simulink model "New_Dstatcom_model"  (R2023a)
settings: Solver=VariableStepAuto  StartTime=0.0  StopTime=0.5  RelTol=1e-3
libraries: spsSeriesRLCBranchLib x10, spsThreePhaseBreakerLib x9, spsThreePhaseSeriesRLCLoadLib x9, spsIGBTDiodeLib x6, spsPower3phInstantaneousLib x3, fuzblock x3, spsThreePhaseVIMeasurementLib x3, spsAlphaBetaZerotodq0Lib x2, spsabctodq0Lib x2, slpidlib x1, simulink x1, spsdq0toabcLib x1
settings Model: Creator=Lenovo  LastModifiedBy=Deepak

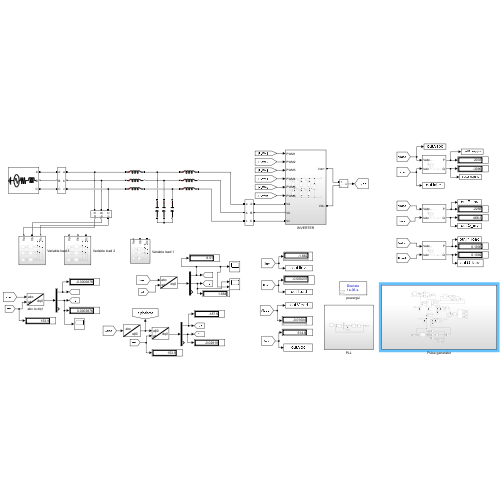
[thumbnail: Simulink's stored preview of the top-level diagram]
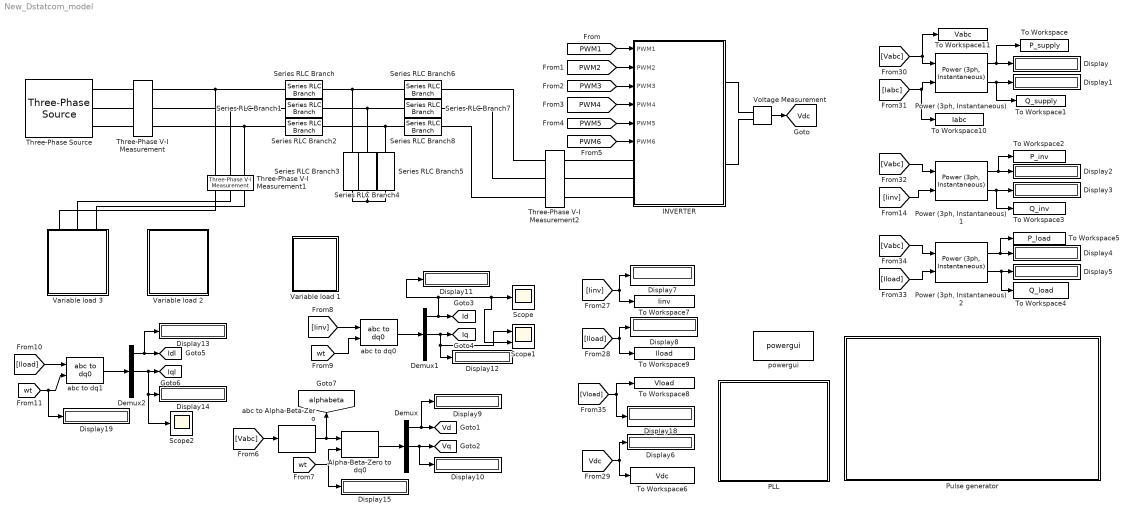
== system New_Dstatcom_model ==
  Alpha-Beta-Zero to dq0 : spsAlphaBetaZerotodq0Lib/Alpha-Beta-Zero to dq0  Alignment=90 degrees behind phase A axis
  Demux : Demux  Outputs=3
  Demux1 : Demux  Outputs=3
  Demux2 : Demux  Outputs=3
  Display{,1..15,18..19} (18 alike) : Display
  INVERTER : Subsystem
  PLL : Subsystem
  "Power (3ph, Instantaneous)" : spsPower3phInstantaneousLib/Power (3ph, Instantaneous)
  "Power (3ph, Instantaneous)1" : spsPower3phInstantaneousLib/Power (3ph, Instantaneous)
  "Power (3ph, Instantaneous)2" : spsPower3phInstantaneousLib/Power (3ph, Instantaneous)
  Pulse generator : Subsystem
  Scope : Scope
  Scope1 : Scope  NumInputPorts=2
  Scope2 : Scope
  Series RLC Branch{,1..2,6..8} (6 alike) : spsSeriesRLCBranchLib/Series RLC Branch  LConnTagsString=__new0  RConnTagsString=__new0  BranchType=L  Resistance=1  Inductance=500e-6  SetiL0=off  InitialCurrent=0  Capacitance=1e-6  Setx0=off  InitialVoltage=0  Measurements=None
  Series RLC Branch3 : spsSeriesRLCBranchLib/Series RLC Branch  LConnTagsString=__new0  RConnTagsString=__new0  BranchType=C  Resistance=1  Inductance=500e-6  SetiL0=off  InitialCurrent=0  Capacitance=100e-6  Setx0=off  InitialVoltage=0  Measurements=None
  Series RLC Branch4 : spsSeriesRLCBranchLib/Series RLC Branch  LConnTagsString=__new0  RConnTagsString=__new0  BranchType=C  Resistance=1  Inductance=500e-6  SetiL0=off  InitialCurrent=0  Capacitance=100e-6  Setx0=off  InitialVoltage=0  Measurements=None
  Series RLC Branch5 : spsSeriesRLCBranchLib/Series RLC Branch  LConnTagsString=__new0  RConnTagsString=__new0  BranchType=C  Resistance=1  Inductance=500e-6  SetiL0=off  InitialCurrent=0  Capacitance=100e-6  Setx0=off  InitialVoltage=0  Measurements=None
  Three-Phase V-I Measurement : spsThreePhaseVIMeasurementLib/Three-Phase V-I Measurement  VoltageMeasurement=phase-to-ground  SetLabelV=on  LabelV=Vabc  Vpu=off  VpuLL=off  CurrentMeasurement=yes  SetLabelI=on  LabelI=Iabc  Ipu=off  Pbase=100e6  Vbase=500e3  OutputType=Complex  PhasorSimulation=off  PSBequivalent=0
  Three-Phase V-I Measurement1 : spsThreePhaseVIMeasurementLib/Three-Phase V-I Measurement  VoltageMeasurement=phase-to-ground  SetLabelV=on  LabelV=Vload  Vpu=off  VpuLL=off  CurrentMeasurement=yes  SetLabelI=on  LabelI=Iload  Ipu=off  Pbase=100e6  Vbase=500e3  OutputType=Complex  PhasorSimulation=off  PSBequivalent=0
  Three-Phase V-I Measurement2 : spsThreePhaseVIMeasurementLib/Three-Phase V-I Measurement  VoltageMeasurement=phase-to-ground  SetLabelV=on  LabelV=Vinv  Vpu=off  VpuLL=off  CurrentMeasurement=yes  SetLabelI=on  LabelI=Iinv  Ipu=off  Pbase=100e6  Vbase=500e3  OutputType=Complex  PhasorSimulation=off  PSBequivalent=0
  Three-Phase Source : spsThreePhaseSourceLib/Three-Phase Source  InternalConnection=Yg  VoltagePhases=off  Voltage=230  PhaseAngle=0  Voltage_phases=[25e3 25e3 25e3]/sqrt(3)  PhaseAngles_phases=[0 -120 +120]  Frequency=50  NonIdealSource=on  SpecifyImpedance=off  Resistance=1e-6  Inductance=1e-6  ShortCircuitLevel=100e6  BaseVoltage=415  XRratio=7  BusType=swing  Pref=10e3  Qref=0  Prefabc=[10e3, 10e3, 10e3]  Qrefabc=[0, 0, 0]  Qmin=-inf  Qmax=inf
  To Workspace : ToWorkspace  VariableName=P_supply  SaveFormat=Timeseries  SampleTime=-1
  To Workspace1 : ToWorkspace  VariableName=Q_supply  SaveFormat=Timeseries  SampleTime=-1
  To Workspace10 : ToWorkspace  VariableName=Iabc  SaveFormat=Timeseries  SampleTime=-1
  To Workspace11 : ToWorkspace  VariableName=Vabc  SaveFormat=Timeseries  SampleTime=-1
  To Workspace2 : ToWorkspace  VariableName=P_inv  SaveFormat=Timeseries  SampleTime=-1
  To Workspace3 : ToWorkspace  VariableName=Q_inv  SaveFormat=Timeseries  SampleTime=-1
  To Workspace4 : ToWorkspace  VariableName=Q_load  SaveFormat=Timeseries  SampleTime=-1
  To Workspace5 : ToWorkspace  VariableName=P_load  SaveFormat=Timeseries  SampleTime=-1
  To Workspace6 : ToWorkspace  VariableName=Vdc  SaveFormat=Timeseries  SampleTime=-1
  To Workspace7 : ToWorkspace  VariableName=Iinv  SaveFormat=Timeseries  SampleTime=-1
  To Workspace8 : ToWorkspace  VariableName=Vload  SaveFormat=Timeseries  SampleTime=-1
  To Workspace9 : ToWorkspace  VariableName=Iload  SaveFormat=Timeseries  SampleTime=-1
  Variable load 1 : Subsystem
  Variable load 2 : Subsystem
  Variable load 3 : Subsystem
  Voltage Measurement : spsVoltageMeasurementLib/Voltage Measurement  PhasorSimulation=off  OutputType=Complex  PSBequivalent=0
  abc to Alpha-Beta-Zero : spsabctoAlphaBetaZeroLib/abc to Alpha-Beta-Zero
  abc to dq0 : spsabctodq0Lib/abc to dq0  Alignment=90 degrees behind phase A axis
  abc to dq1 : spsabctodq0Lib/abc to dq0  Alignment=90 degrees behind phase A axis
  powergui : sps_lib/powergui  Priority=1  SimulationMode=Discrete  SampleTime=1e-6  frequency=60  Iterations=50  frequencyindice=0  Pbase=100e6  ErrMax=1e-4  UnitsV=kV  UnitsW=MW  buscounter=0  FunctionMessages=off  echomessages=off  EnableUseOfTLC=off  CurrentSourceSwitches=off  DisableSnubberDevices=off  DisableRonSwitches=off  DisableVfSwitches=off  DisplayEquations=off  AutomaticDiscreteSolvers=off  SolverType=Tustin/Backward Euler (TBE)  Interpol=off  ExternalGateDelay=off  methode=off  Ts=100  x0status=blocks  SPID=on  SwTol=0  HookPort=off  NonlinearTolerance=1e-4  nMaxIteration=100  ContinueOnMaxIteration=off  RestoreLinks=warning  ResistiveCurrentMeasurement=off  Frange=[0:2:500]  Ylog=off  Xlog=on  ShowGrid=off  save=off  variable=ZData  structure=0  ZoomFFT=off  StartTime=0.0  cycles=1  DisplayStyle=1  fundamental=60  FreqAxis=off  MaxFrequency=1000  frequencyindicesteady=1  RmsSteady=1  display=off
  tag scope: Id=global, Idl=global, Iq=global, Iql=global, Vd=global, Vdc=global, Vq=global, alphabeta=global
  wires:
  [PWM1] -> INVERTER/1(PWM1)
  [PWM2] -> INVERTER/2(PWM2)
  [PWM3] -> INVERTER/3(PWM3)
  [PWM4] -> INVERTER/4(PWM4)
  [PWM5] -> INVERTER/5(PWM5)
  [PWM6] -> INVERTER/6(PWM6)
  Voltage Measurement/1 -> [Vdc]
  [Vabc] -> abc to Alpha-Beta-Zero/1
  abc to Alpha-Beta-Zero/1 -> Alpha-Beta-Zero to dq0/1, [alphabeta]
  [wt] -> Display15/1, Alpha-Beta-Zero to dq0/2
  Alpha-Beta-Zero to dq0/1 -> Demux/1
  Demux/1 -> Display9/1, [Vd]
  Demux/2 -> Display10/1, [Vq]
  [Iinv] -> abc to dq0/1
  [wt] -> abc to dq0/2
  Demux1/2 -> Scope1/1, Display12/1, [Iq]
  Demux1/1 -> Display11/1, Scope1/2, Scope/1, [Id]
  abc to dq0/1 -> Demux1/1
  Demux2/1 -> Display13/1, [Idl]
  Demux2/2 -> Scope2/1, Display14/1, [Iql]
  [wt] -> Display19/1, abc to dq1/2
  abc to dq1/1 -> Demux2/1
  [Iload] -> abc to dq1/1
  "Power (3ph, Instantaneous)"/1 -> To Workspace/1, Display/1
  "Power (3ph, Instantaneous)"/2 -> To Workspace1/1, Display1/1
  [Vabc] -> To Workspace11/1, "Power (3ph, Instantaneous)"/1
  [Iabc] -> To Workspace10/1, "Power (3ph, Instantaneous)"/2
  [Vabc] -> "Power (3ph, Instantaneous)1"/1
  "Power (3ph, Instantaneous)1"/1 -> To Workspace2/1, Display2/1
  "Power (3ph, Instantaneous)1"/2 -> To Workspace3/1, Display3/1
  [Vabc] -> "Power (3ph, Instantaneous)2"/1
  "Power (3ph, Instantaneous)2"/1 -> To Workspace5/1, Display4/1
  "Power (3ph, Instantaneous)2"/2 -> To Workspace4/1, Display5/1
  [Iinv] -> "Power (3ph, Instantaneous)1"/2
  [Iload] -> "Power (3ph, Instantaneous)2"/2
  [Iload] -> To Workspace9/1, Display8/1
  [Iinv] -> To Workspace7/1, Display7/1
  [Vdc] -> Display6/1, To Workspace6/1
  [Vload] -> To Workspace8/1, Display18/1
  connections:
  Three-Phase Source/RConn1 -- Three-Phase V-I Measurement/LConn1
  Three-Phase Source/RConn2 -- Three-Phase V-I Measurement/LConn2
  Three-Phase Source/RConn3 -- Three-Phase V-I Measurement/LConn3
  Series RLC Branch/LConn1 -- Three-Phase V-I Measurement/RConn1 -- Three-Phase V-I Measurement1/LConn1
  Series RLC Branch1/LConn1 -- Three-Phase V-I Measurement/RConn2 -- Three-Phase V-I Measurement1/LConn2
  Series RLC Branch2/LConn1 -- Three-Phase V-I Measurement/RConn3 -- Three-Phase V-I Measurement1/LConn3
  Series RLC Branch3/RConn1 -- Series RLC Branch4/RConn1 -- Series RLC Branch5/RConn1
  Series RLC Branch/RConn1 -- Series RLC Branch6/LConn1 -- Series RLC Branch3/LConn1
  Series RLC Branch1/RConn1 -- Series RLC Branch7/LConn1 -- Series RLC Branch4/LConn1
  Series RLC Branch2/RConn1 -- Series RLC Branch8/LConn1 -- Series RLC Branch5/LConn1
  Three-Phase V-I Measurement2/RConn1 -- Series RLC Branch6/RConn1
  Series RLC Branch7/RConn1 -- Three-Phase V-I Measurement2/RConn2
  Series RLC Branch8/RConn1 -- Three-Phase V-I Measurement2/RConn3
  INVERTER/LConn1 -- Three-Phase V-I Measurement2/LConn1
  INVERTER/LConn2 -- Three-Phase V-I Measurement2/LConn2
  INVERTER/LConn3 -- Three-Phase V-I Measurement2/LConn3
  Voltage Measurement/LConn1 -- INVERTER/RConn1
  Voltage Measurement/LConn2 -- INVERTER/RConn2
  Variable load 3/LConn1 -- Three-Phase V-I Measurement1/RConn1
  Variable load 3/LConn2 -- Three-Phase V-I Measurement1/RConn2
  Variable load 3/LConn3 -- Three-Phase V-I Measurement1/RConn3

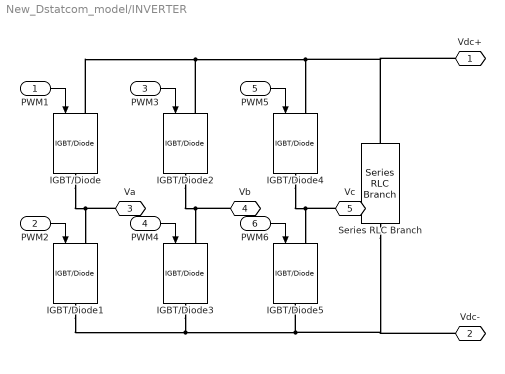
== system New_Dstatcom_model/INVERTER ==
  PWM1 : Inport
  PWM2 : Inport  Port=2
  PWM3 : Inport  Port=3
  PWM4 : Inport  Port=4
  PWM5 : Inport  Port=5
  PWM6 : Inport  Port=6
  IGBT/Diode{,1..5} (6 alike) : spsIGBTDiodeLib/IGBT//Diode  Ron=1e-3  Rs=1e5  Cs=inf  Measurements=off
  Series RLC Branch : spsSeriesRLCBranchLib/Series RLC Branch  LConnTagsString=__new0  RConnTagsString=__new0  BranchType=RC  Resistance=1e-3  Inductance=1e-3  SetiL0=off  InitialCurrent=0  Capacitance=5600e-6  Setx0=off  InitialVoltage=0  Measurements=None
  Vdc+ : PMIOPort  Side=Right
  Vdc- : PMIOPort  Port=2  Side=Right
  Va : PMIOPort  Port=3  Side=Left
  Vb : PMIOPort  Port=4  Side=Left
  Vc : PMIOPort  Port=5  Side=Left
  wires:
  PWM1/1 -> IGBT/Diode/1
  PWM5/1 -> IGBT/Diode4/1
  PWM2/1 -> IGBT/Diode1/1
  PWM4/1 -> IGBT/Diode3/1
  PWM6/1 -> IGBT/Diode5/1
  PWM3/1 -> IGBT/Diode2/1
  connections:
  IGBT/Diode/LConn1 -- Vdc+/RConn1 -- Series RLC Branch/LConn1 -- IGBT/Diode4/LConn1 -- IGBT/Diode2/LConn1
  IGBT/Diode4/RConn1 -- Vc/RConn1 -- IGBT/Diode5/LConn1
  IGBT/Diode2/RConn1 -- Vb/RConn1 -- IGBT/Diode3/LConn1
  IGBT/Diode/RConn1 -- Va/RConn1 -- IGBT/Diode1/LConn1
  IGBT/Diode1/RConn1 -- IGBT/Diode3/RConn1 -- Vdc-/RConn1 -- Series RLC Branch/RConn1 -- IGBT/Diode5/RConn1

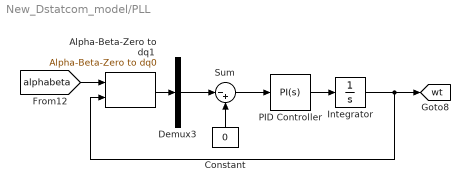
== system New_Dstatcom_model/PLL ==
  Alpha-Beta-Zero to dq1 : spsAlphaBetaZerotodq0Lib/Alpha-Beta-Zero to dq0  Alignment=90 degrees behind phase A axis
  Constant : Constant  Value=0
  Demux3 : Demux  Outputs=3
  Integrator : Integrator
  PID Controller : slpidlib/PID Controller  Controller=PI  Form=Parallel  TimeDomain=Continuous-time  UseExternalTs=off  SampleTime=-1  IntegratorMethod=Forward Euler  FilterMethod=Forward Euler  ControllerParametersSource=internal  P=10  I=50000  UseKiTs=off  D=0  N=100  UseFilter=on  TunerSelectOption=Transfer Function Based (PID Tuner App)  InitialConditionSource=internal  InitialConditionForIntegrator=0  InitialConditionForFilter=0  DifferentiatorICPrevScaledInput=0  ExternalReset=none  TrackingMode=off  Kt=1  LimitOutput=off  SatLimitsSource=internal  UpperSaturationLimit=inf  LowerSaturationLimit=-inf  LinearizeAsGain=on  AntiWindupMode=none  Kb=1  LimitIntegrator=off  UpperIntegratorSaturationLimit=inf  LowerIntegratorSaturationLimit=-inf  POutMin=[]  POutMax=[]  IOutMin=[]  IOutMax=[]  DOutMin=[]  DOutMax=[]  NOutMin=[]  NOutMax=[]  SumOutMin=[]  SumOutMax=[]  SaturationOutMin=[]  SaturationOutMax=[]  PParamMin=[]  PParamMax=[]  IParamMin=[]  IParamMax=[]  DParamMin=[]  DParamMax=[]  NParamMin=[]  NParamMax=[]  KbParamMin=[]  KbParamMax=[]  KtParamMin=[]  KtParamMax=[]  KbOutMin=[]  KbOutMax=[]  KtOutMin=[]  KtOutMax=[]  IntegratorOutMin=[]  IntegratorOutMax=[]  FilterOutMin=[]  FilterOutMax=[]  SumI1OutMin=[]  SumI1OutMax=[]  SumI2OutMin=[]  SumI2OutMax=[]  SumI3OutMin=[]  SumI3OutMax=[]  SumI4OutMin=[]  SumI4OutMax=[]  SumDOutMin=[]  SumDOutMax=[]  DifferentiatorOutMin=[]  DifferentiatorOutMax=[]  FilterDiffOutCoefMin=[]  FilterDiffOutCoefMax=[]  ReciprocalOutMin=[]  ReciprocalOutMax=[]  SumDenOutMin=[]  SumDenOutMax=[]  SumNumOutMin=[]  SumNumOutMax=[]  DivideOutMin=[]  DivideOutMax=[]  UdiffTsProdOutMin=[]  UdiffTsProdOutMax=[]  NTsProdOutMin=[]  NTsProdOutMax=[]  UintegralTsProdOutMin=[]  UintegralTsProdOutMax=[]  UngainTsProdOutMin=[]  UngainTsProdOutMax=[]  ClampingZeroOutDataTypeStr=Inherit: Inherit via back propagation  ClampingZeroOutMin=[]  ClampingZeroOutMax=[]  FilterDenConstantOutDataTypeStr=Inherit: Inherit via back propagation  FilterDenConstantOutMin=[]  FilterDenConstantOutMax=[]  PCopyOutDataTypeStr=Inherit: Inherit via back propagation  PCopyOutMin=[]  PCopyOutMax=[]  NCopyOutDataTypeStr=Inherit: Inherit via back propagation  NCopyOutMin=[]  NCopyOutMax=[]  IntegratorContinuousStateAttributes=''  IntegratorStateMustResolveToSignalObject=off  IntegratorRTWStateStorageClass=Auto  FilterContinuousStateAttributes=''  FilterStateMustResolveToSignalObject=off  FilterRTWStateStorageClass=Auto  ParallelPVariant=InternalParameters  IdealPVariant=Disabled  IVariant=InternalParameters  DVariant=Disabled  IntegratorVariant=Continuous  SatVariant=Disabled  AWVariant=Passthrough  PCopyVariant=Disabled  TRVariant=Disabled  FdbkBlocksVariant=Forward  IdealPFdbkVariant=Disabled  SatFdbkVariant=Disabled  DerivativeFilterVariant=Disabled  NVariant=Disabled  NCopyVariant=Disabled_SignalSpec  FilterICVariant=Disabled  IntegratorICVariant=InternalICs  ExternalResetVariant=Disabled  TRSumVariant=Passthrough  SumFdbkVariant=Disabled  SumVariant=Sum_PI  TsampFilterVariant=InternalTs  TsampNgainVariant=Passthrough  TsampIntegralVariant=Disabled_SignalSpec  ExternalSaturationOutDataTypeStr=Inherit: Same as second input
  Sum : Sum  Inputs=|-+
  tag scope: wt=global
  wires:
  [alphabeta] -> Alpha-Beta-Zero to dq1/1
  PID Controller/1 -> Integrator/1
  Constant/1 -> Sum/2
  Alpha-Beta-Zero to dq1/1 -> Demux3/1
  Integrator/1 -> [wt], Alpha-Beta-Zero to dq1/2
  Sum/1 -> PID Controller/1
  Demux3/2 -> Sum/1

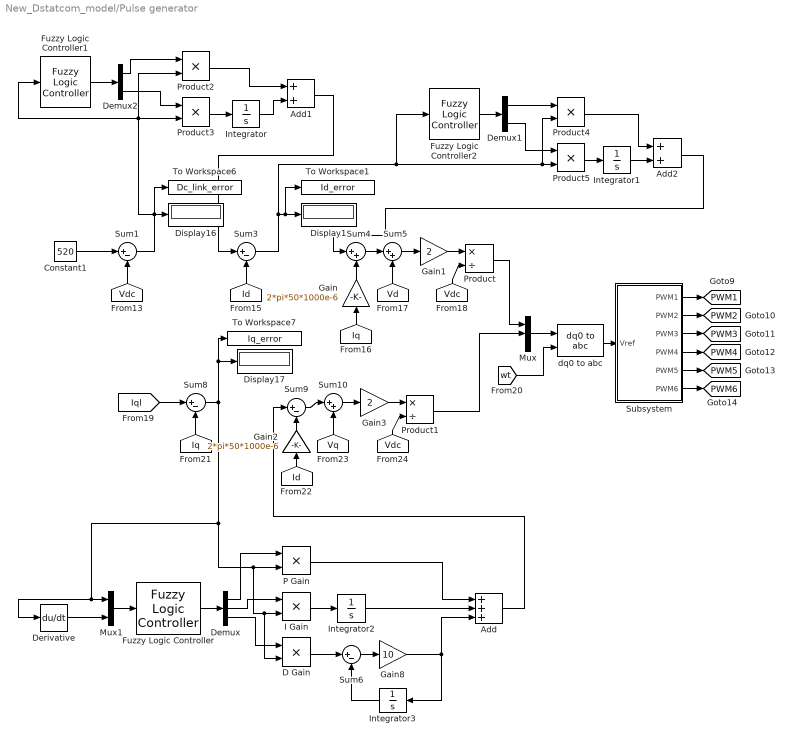
== system New_Dstatcom_model/Pulse generator ==
  Add : Sum  Inputs=+++
  Add1 : Sum
  Add2 : Sum
  Constant1 : Constant  Value=520
  D Gain : Product
  Demux : Demux  Outputs=3
  Demux1 : Demux  Outputs=2
  Demux2 : Demux  Outputs=2
  Derivative : Derivative
  Display1 : Display
  Display16 : Display
  Display17 : Display
  Fuzzy Logic Controller : fuzblock/Fuzzy Logic  Controller  FIS=Npid  OutputSampleNumber=101  DataType=double  FuzzifiedInputs=off  RuleFiringStrengths=off  RuleOutputs=off  AggregatedOutputs=off  SimulateUsing=Interpreted execution  OutOfRangeInputValueMessage=warning  NoRuleFiredMessage=warning  EmptyOutputFuzzySetMessage=warning
  Fuzzy Logic Controller1 : fuzblock/Fuzzy Logic  Controller  FIS=pi1  OutputSampleNumber=101  DataType=double  FuzzifiedInputs=off  RuleFiringStrengths=off  RuleOutputs=off  AggregatedOutputs=off  SimulateUsing=Interpreted execution  OutOfRangeInputValueMessage=warning  NoRuleFiredMessage=warning  EmptyOutputFuzzySetMessage=warning
  Fuzzy Logic Controller2 : fuzblock/Fuzzy Logic  Controller  FIS=pi2  OutputSampleNumber=101  DataType=double  FuzzifiedInputs=off  RuleFiringStrengths=off  RuleOutputs=off  AggregatedOutputs=off  SimulateUsing=Interpreted execution  OutOfRangeInputValueMessage=warning  NoRuleFiredMessage=warning  EmptyOutputFuzzySetMessage=warning
  Gain : Gain  Gain=2*pi*50*1000e-6
  Gain1 : Gain  Gain=2
  Gain2 : Gain  Gain=2*pi*50*1000e-6
  Gain3 : Gain  Gain=2
  Gain8 : Gain  Gain=10
  I Gain : Product
  Integrator{,1..3} (4 alike) : Integrator
  Mux : Mux  Inputs=3
  Mux1 : Mux  Inputs=2
  P Gain : Product
  Product : Product  Inputs=*/
  Product1 : Product  Inputs=*/
  Product{2..5} (4 alike) : Product
  Subsystem : Subsystem
  Sum{1,3,6,8..9} (5 alike) : Sum  Inputs=|+-
  Sum10 : Sum  Inputs=|++
  Sum4 : Sum  Inputs=|++
  Sum5 : Sum  Inputs=|++
  To Workspace1 : ToWorkspace  VariableName=Id_error  SaveFormat=Timeseries  SampleTime=-1
  To Workspace6 : ToWorkspace  VariableName=Dc_link_error  SaveFormat=Timeseries  SampleTime=-1
  To Workspace7 : ToWorkspace  VariableName=Iq_error  SaveFormat=Timeseries  SampleTime=-1
  dq0 to abc : spsdq0toabcLib/dq0 to abc  Alignment=90 degrees behind phase A axis
  tag scope: PWM1=global, PWM2=global, PWM3=global, PWM4=global, PWM5=global, PWM6=global
  wires:
  Gain/1 -> Sum4/2
  Sum4/1 -> Sum5/1
  [Vdc] -> Sum1/2
  [wt] -> dq0 to abc/2
  Subsystem/2(PWM2) -> [PWM2]
  [Vdc] -> Product/2
  Subsystem/6(PWM6) -> [PWM6]
  Sum5/1 -> Gain1/1
  Sum8/1 -> D Gain/2, I Gain/2, P Gain/2, Derivative/1, Mux1/1, To Workspace7/1, Display17/1
  [Vdc] -> Product1/2
  Product/1 -> Mux/1
  Gain2/1 -> Sum9/2
  Constant1/1 -> Sum1/1
  Sum10/1 -> Gain3/1
  Mux/1 -> dq0 to abc/1
  [Vd] -> Sum5/2
  Gain3/1 -> Product1/1
  Subsystem/3(PWM3) -> [PWM3]
  [Id] -> Gain2/1
  Sum3/1 -> Fuzzy Logic Controller2/1, Product4/2, Product5/2, To Workspace1/1, Display1/1
  Subsystem/5(PWM5) -> [PWM5]
  dq0 to abc/1 -> Subsystem/1(Vref)
  [Iq] -> Sum8/2
  Subsystem/1(PWM1) -> [PWM1]
  Product1/1 -> Mux/2
  Sum9/1 -> Sum10/1
  Gain1/1 -> Product/1
  Subsystem/4(PWM4) -> [PWM4]
  [Id] -> Sum3/2
  [Iq] -> Gain/1
  [Vq] -> Sum10/2
  P Gain/1 -> Add/1
  Integrator2/1 -> Add/2
  I Gain/1 -> Integrator2/1
  Product3/1 -> Integrator/1
  Integrator/1 -> Add1/2
  Product2/1 -> Add1/1
  Product5/1 -> Integrator1/1
  Product4/1 -> Add2/1
  Integrator1/1 -> Add2/2
  Sum1/1 -> Fuzzy Logic Controller1/1, Product3/2, Product2/2, Display16/1, To Workspace6/1
  Demux2/1 -> Product2/1
  Demux2/2 -> Product3/1
  [Iql] -> Sum8/1
  Add2/1 -> Sum4/1
  Derivative/1 -> Mux1/2
  Fuzzy Logic Controller/1 -> Demux/1
  Demux1/1 -> Product4/1
  Demux1/2 -> Product5/1
  Fuzzy Logic Controller2/1 -> Demux1/1
  Fuzzy Logic Controller1/1 -> Demux2/1
  Demux/1 -> P Gain/1
  Demux/2 -> I Gain/1
  Demux/3 -> D Gain/1
  D Gain/1 -> Sum6/1
  Sum6/1 -> Gain8/1
  Gain8/1 -> Integrator3/1, Add/3
  Integrator3/1 -> Sum6/2
  Mux1/1 -> Fuzzy Logic Controller/1
  Add1/1 -> Sum3/1
  Add/1 -> Sum9/1

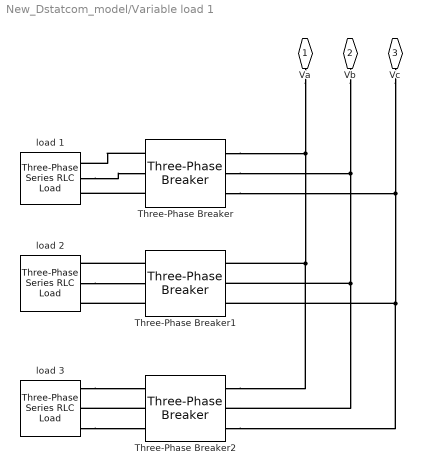
== system New_Dstatcom_model/Variable load 1 ==
  Three-Phase Breaker : spsThreePhaseBreakerLib/Three-Phase Breaker  InitialState=open  SwitchA=on  SwitchB=on  SwitchC=on  SwitchTimes="[0  0.35]"  External=off  BreakerResistance=0.01  SnubberResistance=1e6  SnubberCapacitance=inf  Measurements=None
  Three-Phase Breaker1 : spsThreePhaseBreakerLib/Three-Phase Breaker  InitialState=open  SwitchA=on  SwitchB=on  SwitchC=on  SwitchTimes="[0.1  0.3]"  External=off  BreakerResistance=0.01  SnubberResistance=1e6  SnubberCapacitance=inf  Measurements=None
  Three-Phase Breaker2 : spsThreePhaseBreakerLib/Three-Phase Breaker  InitialState=open  SwitchA=on  SwitchB=on  SwitchC=on  SwitchTimes="[0.2  0.3]"  External=off  BreakerResistance=0.01  SnubberResistance=1e6  SnubberCapacitance=inf  Measurements=None
  load 1 : spsThreePhaseSeriesRLCLoadLib/Three-Phase Series RLC Load  LConnTagsString=A|B|C  Configuration=Y (grounded)  NominalVoltage=230  Vabc=[1e3 1e3 1e3]  Vabcp=[1e3 1e3 1e3]  NominalFrequency=50  UnbalancedPower=off  ActivePower=5e3  InductivePower=10e3  CapacitivePower=0  Pabc=[10e3 9e3 11e3]  QLabc=[100 90 110]  QCabc=[100 90 110]  Pabcp=[10e3 9e3 11e3]  QLabcp=[100 90 110]  QCabcp=[100 90 110]  Measurements=None  LoadType=constant PQ
  load 2 : spsThreePhaseSeriesRLCLoadLib/Three-Phase Series RLC Load  LConnTagsString=A|B|C  Configuration=Y (grounded)  NominalVoltage=230  Vabc=[1e3 1e3 1e3]  Vabcp=[1e3 1e3 1e3]  NominalFrequency=50  UnbalancedPower=off  ActivePower=7e3  InductivePower=25e3  CapacitivePower=0  Pabc=[10e3 9e3 11e3]  QLabc=[100 90 110]  QCabc=[100 90 110]  Pabcp=[10e3 9e3 11e3]  QLabcp=[100 90 110]  QCabcp=[100 90 110]  Measurements=None  LoadType=constant PQ
  load 3 : spsThreePhaseSeriesRLCLoadLib/Three-Phase Series RLC Load  LConnTagsString=A|B|C  Configuration=Y (grounded)  NominalVoltage=230  Vabc=[1e3 1e3 1e3]  Vabcp=[1e3 1e3 1e3]  NominalFrequency=50  UnbalancedPower=off  ActivePower=15e3  InductivePower=70e3  CapacitivePower=0  Pabc=[10e3 9e3 11e3]  QLabc=[100 90 110]  QCabc=[100 90 110]  Pabcp=[10e3 9e3 11e3]  QLabcp=[100 90 110]  QCabcp=[100 90 110]  Measurements=None  LoadType=constant PQ
  Va : PMIOPort  Side=Left
  Vb : PMIOPort  Port=2  Side=Left
  Vc : PMIOPort  Port=3  Side=Left
  connections:
  load 1/LConn2 -- Three-Phase Breaker/LConn2
  Three-Phase Breaker1/LConn3 -- load 2/LConn3
  load 3/LConn1 -- Three-Phase Breaker2/LConn1
  Three-Phase Breaker/LConn1 -- load 1/LConn1
  Three-Phase Breaker/LConn3 -- load 1/LConn3
  Three-Phase Breaker1/LConn1 -- load 2/LConn1
  Three-Phase Breaker/RConn3 -- Vc/RConn1 -- Three-Phase Breaker2/RConn3 -- Three-Phase Breaker1/RConn3
  load 2/LConn2 -- Three-Phase Breaker1/LConn2
  load 3/LConn3 -- Three-Phase Breaker2/LConn3
  Three-Phase Breaker2/LConn2 -- load 3/LConn2
  Three-Phase Breaker/RConn2 -- Vb/RConn1 -- Three-Phase Breaker2/RConn2 -- Three-Phase Breaker1/RConn2
  Three-Phase Breaker/RConn1 -- Va/RConn1 -- Three-Phase Breaker2/RConn1 -- Three-Phase Breaker1/RConn1

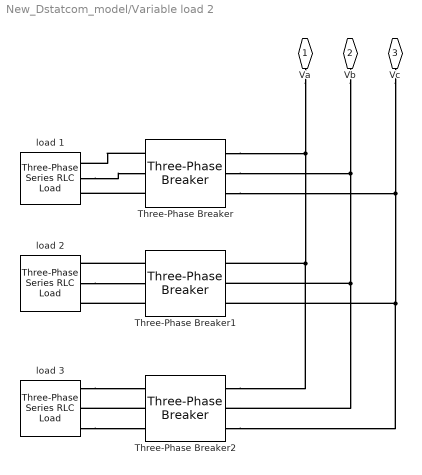
== system New_Dstatcom_model/Variable load 2 ==
  Three-Phase Breaker : spsThreePhaseBreakerLib/Three-Phase Breaker  InitialState=open  SwitchA=on  SwitchB=on  SwitchC=on  SwitchTimes="[0  0.35]"  External=off  BreakerResistance=0.01  SnubberResistance=1e6  SnubberCapacitance=inf  Measurements=None
  Three-Phase Breaker1 : spsThreePhaseBreakerLib/Three-Phase Breaker  InitialState=open  SwitchA=on  SwitchB=on  SwitchC=on  SwitchTimes="[0.1  0.3]"  External=off  BreakerResistance=0.01  SnubberResistance=1e6  SnubberCapacitance=inf  Measurements=None
  Three-Phase Breaker2 : spsThreePhaseBreakerLib/Three-Phase Breaker  InitialState=open  SwitchA=on  SwitchB=on  SwitchC=on  SwitchTimes="[0.2  0.3]"  External=off  BreakerResistance=0.01  SnubberResistance=1e6  SnubberCapacitance=inf  Measurements=None
  load 1 : spsThreePhaseSeriesRLCLoadLib/Three-Phase Series RLC Load  LConnTagsString=A|B|C  Configuration=Y (grounded)  NominalVoltage=230  Vabc=[1e3 1e3 1e3]  Vabcp=[1e3 1e3 1e3]  NominalFrequency=50  UnbalancedPower=off  ActivePower=5e3  InductivePower=10e3  CapacitivePower=0  Pabc=[10e3 9e3 11e3]  QLabc=[100 90 110]  QCabc=[100 90 110]  Pabcp=[10e3 9e3 11e3]  QLabcp=[100 90 110]  QCabcp=[100 90 110]  Measurements=None  LoadType=constant PQ
  load 2 : spsThreePhaseSeriesRLCLoadLib/Three-Phase Series RLC Load  LConnTagsString=A|B|C  Configuration=Y (grounded)  NominalVoltage=230  Vabc=[1e3 1e3 1e3]  Vabcp=[1e3 1e3 1e3]  NominalFrequency=50  UnbalancedPower=off  ActivePower=7e3  InductivePower=25e3  CapacitivePower=0  Pabc=[10e3 9e3 11e3]  QLabc=[100 90 110]  QCabc=[100 90 110]  Pabcp=[10e3 9e3 11e3]  QLabcp=[100 90 110]  QCabcp=[100 90 110]  Measurements=None  LoadType=constant PQ
  load 3 : spsThreePhaseSeriesRLCLoadLib/Three-Phase Series RLC Load  LConnTagsString=A|B|C  Configuration=Y (grounded)  NominalVoltage=230  Vabc=[1e3 1e3 1e3]  Vabcp=[1e3 1e3 1e3]  NominalFrequency=50  UnbalancedPower=off  ActivePower=15e3  InductivePower=70e3  CapacitivePower=0  Pabc=[10e3 9e3 11e3]  QLabc=[100 90 110]  QCabc=[100 90 110]  Pabcp=[10e3 9e3 11e3]  QLabcp=[100 90 110]  QCabcp=[100 90 110]  Measurements=None  LoadType=constant PQ
  Va : PMIOPort  Side=Left
  Vb : PMIOPort  Port=2  Side=Left
  Vc : PMIOPort  Port=3  Side=Left
  connections:
  load 1/LConn2 -- Three-Phase Breaker/LConn2
  Three-Phase Breaker1/LConn3 -- load 2/LConn3
  load 3/LConn1 -- Three-Phase Breaker2/LConn1
  Three-Phase Breaker/LConn1 -- load 1/LConn1
  Three-Phase Breaker/LConn3 -- load 1/LConn3
  Three-Phase Breaker1/LConn1 -- load 2/LConn1
  Three-Phase Breaker/RConn3 -- Vc/RConn1 -- Three-Phase Breaker2/RConn3 -- Three-Phase Breaker1/RConn3
  load 2/LConn2 -- Three-Phase Breaker1/LConn2
  load 3/LConn3 -- Three-Phase Breaker2/LConn3
  Three-Phase Breaker2/LConn2 -- load 3/LConn2
  Three-Phase Breaker/RConn2 -- Vb/RConn1 -- Three-Phase Breaker2/RConn2 -- Three-Phase Breaker1/RConn2
  Three-Phase Breaker/RConn1 -- Va/RConn1 -- Three-Phase Breaker2/RConn1 -- Three-Phase Breaker1/RConn1

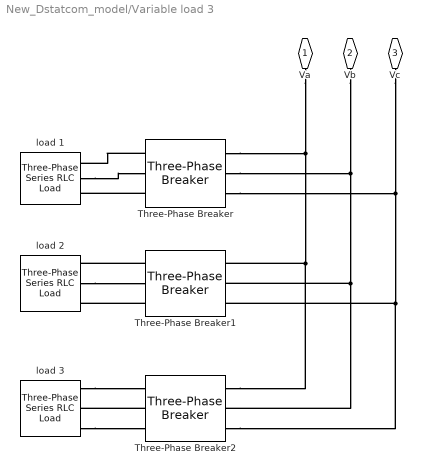
== system New_Dstatcom_model/Variable load 3 ==
  Three-Phase Breaker : spsThreePhaseBreakerLib/Three-Phase Breaker  InitialState=open  SwitchA=on  SwitchB=on  SwitchC=on  SwitchTimes="[0  0.35]"  External=off  BreakerResistance=0.01  SnubberResistance=1e6  SnubberCapacitance=inf  Measurements=None
  Three-Phase Breaker1 : spsThreePhaseBreakerLib/Three-Phase Breaker  InitialState=open  SwitchA=on  SwitchB=on  SwitchC=on  SwitchTimes="[0.1  0.3]"  External=off  BreakerResistance=0.01  SnubberResistance=1e6  SnubberCapacitance=inf  Measurements=None
  Three-Phase Breaker2 : spsThreePhaseBreakerLib/Three-Phase Breaker  InitialState=open  SwitchA=on  SwitchB=on  SwitchC=on  SwitchTimes="[0.2  0.3]"  External=off  BreakerResistance=0.01  SnubberResistance=1e6  SnubberCapacitance=inf  Measurements=None
  load 1 : spsThreePhaseSeriesRLCLoadLib/Three-Phase Series RLC Load  LConnTagsString=A|B|C  Configuration=Y (grounded)  NominalVoltage=230  Vabc=[1e3 1e3 1e3]  Vabcp=[1e3 1e3 1e3]  NominalFrequency=50  UnbalancedPower=off  ActivePower=10e3  InductivePower=0  CapacitivePower=7e3  Pabc=[10e3 9e3 11e3]  QLabc=[100 90 110]  QCabc=[100 90 110]  Pabcp=[10e3 9e3 11e3]  QLabcp=[100 90 110]  QCabcp=[100 90 110]  Measurements=None  LoadType=constant PQ
  load 2 : spsThreePhaseSeriesRLCLoadLib/Three-Phase Series RLC Load  LConnTagsString=A|B|C  Configuration=Y (grounded)  NominalVoltage=230  Vabc=[1e3 1e3 1e3]  Vabcp=[1e3 1e3 1e3]  NominalFrequency=50  UnbalancedPower=off  ActivePower=7e3  InductivePower=0  CapacitivePower=20e3  Pabc=[10e3 9e3 11e3]  QLabc=[100 90 110]  QCabc=[100 90 110]  Pabcp=[10e3 9e3 11e3]  QLabcp=[100 90 110]  QCabcp=[100 90 110]  Measurements=None  LoadType=constant PQ
  load 3 : spsThreePhaseSeriesRLCLoadLib/Three-Phase Series RLC Load  LConnTagsString=A|B|C  Configuration=Y (grounded)  NominalVoltage=230  Vabc=[1e3 1e3 1e3]  Vabcp=[1e3 1e3 1e3]  NominalFrequency=50  UnbalancedPower=off  ActivePower=15e3  InductivePower=0  CapacitivePower=30e3  Pabc=[10e3 9e3 11e3]  QLabc=[100 90 110]  QCabc=[100 90 110]  Pabcp=[10e3 9e3 11e3]  QLabcp=[100 90 110]  QCabcp=[100 90 110]  Measurements=None  LoadType=constant PQ
  Va : PMIOPort  Side=Left
  Vb : PMIOPort  Port=2  Side=Left
  Vc : PMIOPort  Port=3  Side=Left
  connections:
  load 1/LConn2 -- Three-Phase Breaker/LConn2
  Three-Phase Breaker1/LConn3 -- load 2/LConn3
  load 3/LConn1 -- Three-Phase Breaker2/LConn1
  Three-Phase Breaker/LConn1 -- load 1/LConn1
  Three-Phase Breaker/LConn3 -- load 1/LConn3
  Three-Phase Breaker1/LConn1 -- load 2/LConn1
  Three-Phase Breaker/RConn3 -- Vc/RConn1 -- Three-Phase Breaker2/RConn3 -- Three-Phase Breaker1/RConn3
  load 2/LConn2 -- Three-Phase Breaker1/LConn2
  load 3/LConn3 -- Three-Phase Breaker2/LConn3
  Three-Phase Breaker2/LConn2 -- load 3/LConn2
  Three-Phase Breaker/RConn2 -- Vb/RConn1 -- Three-Phase Breaker2/RConn2 -- Three-Phase Breaker1/RConn2
  Three-Phase Breaker/RConn1 -- Va/RConn1 -- Three-Phase Breaker2/RConn1 -- Three-Phase Breaker1/RConn1

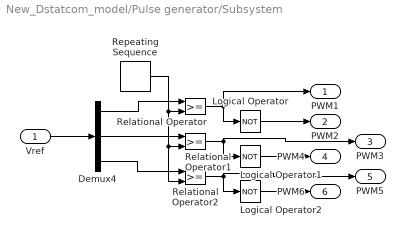
== system New_Dstatcom_model/Pulse generator/Subsystem ==
  Vref : Inport
  Demux4 : Demux  Outputs=3
  Logical Operator : Logic  Operator=NOT  AllPortsSameDT=off  OutDataTypeStr=boolean
  Logical Operator1 : Logic  Operator=NOT  AllPortsSameDT=off  OutDataTypeStr=boolean
  Logical Operator2 : Logic  Operator=NOT  AllPortsSameDT=off  OutDataTypeStr=boolean
  Relational Operator : RelationalOperator  OutDataTypeStr=boolean  RndMeth=Simplest  InputSameDT=off
  Relational Operator1 : RelationalOperator  OutDataTypeStr=boolean  RndMeth=Simplest  InputSameDT=off
  Relational Operator2 : RelationalOperator  OutDataTypeStr=boolean  RndMeth=Simplest  InputSameDT=off
  Repeating Sequence : simulink/Sources/Repeating Sequence  rep_seq_t=[0 0.00005 0.0001]  rep_seq_y=[-1 1 -1]
  PWM1 : Outport
  PWM2 : Outport  Port=2
  PWM3 : Outport  Port=3
  PWM4 : Outport  Port=4
  PWM5 : Outport  Port=5
  PWM6 : Outport  Port=6
  wires:
  Relational Operator2/1 -> PWM5/1, Logical Operator2/1
  Demux4/2 -> Relational Operator1/1
  Relational Operator1/1 -> PWM3/1, Logical Operator1/1
  Repeating Sequence/1 -> Relational Operator2/2, Relational Operator1/2, Relational Operator/2
  Relational Operator/1 -> PWM1/1, Logical Operator/1
  Logical Operator1/1 -> PWM4/1
  Demux4/1 -> Relational Operator/1
  Demux4/3 -> Relational Operator2/1
  Logical Operator/1 -> PWM2/1
  Logical Operator2/1 -> PWM6/1
  Vref/1 -> Demux4/1
